simulink model "sim_yawangle"  (R2022b)
settings: Solver=ode4  StartTime=0.0  StopTime=10.0  FixedStep=1e-3  RelTol=1e-12  EnableMultiTasking=on
libraries: cstblocks x1
settings Model: Creator=Riccardo  LastModifiedBy=tonegas
settings SolverCC: AlgebraicLoopSolver=TrustRegion
settings DataIOCC: LimitDataPoints=on  SaveFormat=Array  SignalLoggingSaveFormat=ModelDataLogs  ReturnWorkspaceOutputs=off
settings OptimizationCC: ExpressionDepthLimit=2147483647  LifeSpan=inf
settings DebuggingCC: UnderspecifiedInitializationDetection=Classic  MergeDetectMultiDrivingBlocksExec=none  SolverPrmCheckMsg=warning  FcnCallInpInsideContextMsg=warning  UnconnectedInputMsg=warning  UnconnectedOutputMsg=warning  UnconnectedLineMsg=warning  StateNameClashWarn=warning  SFUnexpectedBacktrackingDiag=warning  SFNoUnconditionalDefaultTransitionDiag=warning  SFExecutionAtInitializationDiag=none  SFMachineParentedDataDiag=warning  ArithmeticOperatorsInVariantConditions=warning
settings HardwareCC: ProdBitPerPointer=32  ProdBitPerSizeT=32  ProdBitPerPtrDiffT=32  ProdLargestAtomicFloat=None  ProdIntDivRoundTo=Undefined  ProdEndianess=Unspecified  ProdWordSize=32  ProdHWDeviceType=32-bit Generic
settings ModelReferenceCC: EnableRefExpFcnMdlSchedulingChecks=on  PropagateSignalLabelsOutOfModel=off
settings SFSimCC: SimUseLocalCustomCode=off  CustomCodeUndefinedFunction=UseInterfaceOnly
settings RTWCC: RTWUseLocalCustomCode=off
settings CodeAppCC: StateflowObjectComments=on
settings GRTTargetCC: TargetLangStandard=C89/C90 (ANSI)  CombineOutputUpdateFcns=off  GRTInterface=on
settings ConfigComp: CovMetricSettings=dw  CovSaveCumulativeToWorkspaceVar=on  CovSaveSingleToWorkspaceVar=on  CovExternalEMLEnable=off

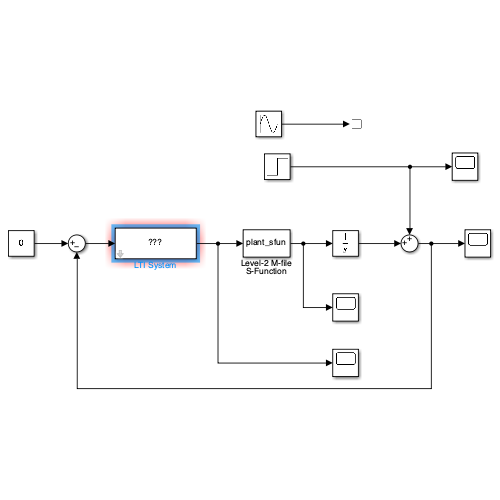
[thumbnail: Simulink's stored preview of the top-level diagram]
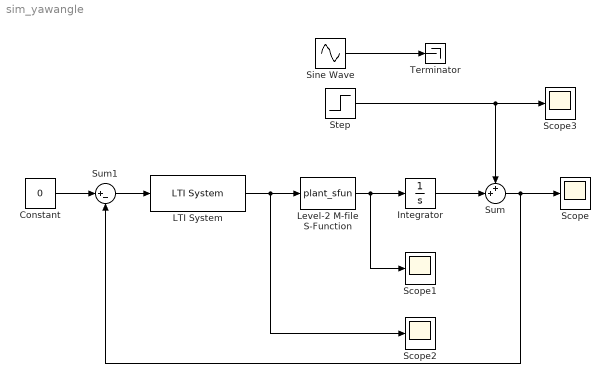
== system sim_yawangle ==
  Constant : Constant  Value=0
  Integrator : Integrator
  LTI System : cstblocks/LTI System  sys=PD  IC=[]
  Level-2 M-file S-Function : M-S-Function  FunctionName=plant_sfun
  Scope{,1..3} (4 alike) : Scope
  Sine Wave : Sin  Amplitude=0.01  Frequency=5  SampleTime=0
  Step : Step  After=0.1  SampleTime=0
  Sum : Sum  Inputs=++|
  Sum1 : Sum  Inputs=|+-
  Terminator : Terminator
  wires:
  Sum1/1 -> LTI System/1
  Sum/1 -> Sum1/2, Scope/1
  Constant/1 -> Sum1/1
  Level-2 M-file S-Function/1 -> Integrator/1, Scope1/1
  Integrator/1 -> Sum/2
  LTI System/1 -> Level-2 M-file S-Function/1, Scope2/1
  Step/1 -> Sum/1, Scope3/1
  Sine Wave/1 -> Terminator/1
